simulink model "SOH_second"  (R2025a)
settings: Solver=VariableStepAuto  StartTime=0.0  StopTime=100  RelTol=1e-3
libraries: nesl_utility x7, fl_lib x5, batt_lib x1, spsDiscreteVariableTimeDelayLib x1, BatteryEstimators x1
settings Model: Creator=aassd  LastModifiedBy=aassd

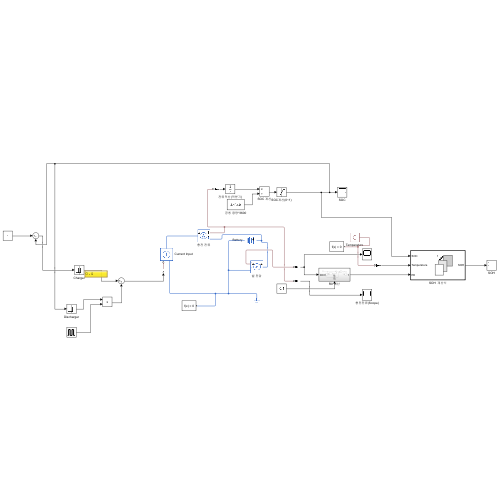
[thumbnail: Simulink's stored preview of the top-level diagram]
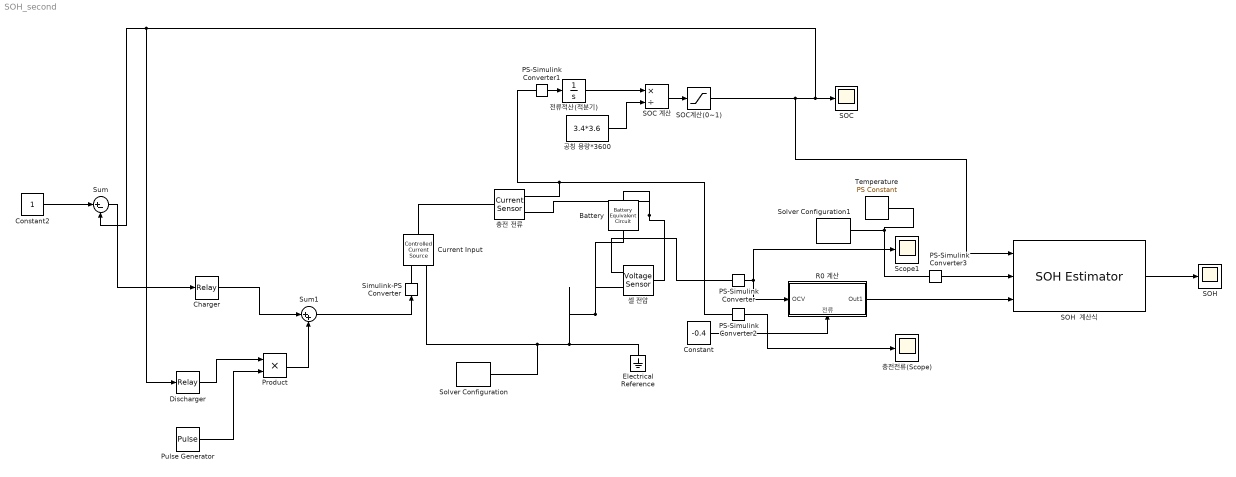
== system SOH_second ==
  Battery : batt_lib/Cells/Battery Equivalent Circuit  BatteryCapacity=3.4 A*hr  ThermalModel=simscape.battery.enum.cells.BatteryThermalModel.ConstantTemperature  ExtrapolationMethod=simscape.enum.extrapolation.linear  SOCBreakpoints=[0, 0.111071, 0.222202, 0.333333, 0.444465, 0.555535, 0.666667, 0.777798, 0.888869]  TemperatureBreakpoints=[273.15, 298.15, 318.15] K  OpenCircuitVoltage=[3.5057, 3.566, 3.6337, 3.7127, 3.9259, 4.0777, 4.1928] V  OpenCircuitVoltageThermal=[4.0405, 4.0578, 4.0648; 3.9374, 3.9475, 3.9556; 3.844, 3.8471, 3.8552; 3.759, 3.7591, 3.7659; 3.671, 3.67, 3.6778; 3.6282, 3.6287, 3.6355; 3.6009, 3.6013, 3.608; 3.5742, 3.5621, 3.5612; 3.4716, 3.3585, 3.3997;] V  VoltageRange=[0, inf] V  HysteresisModel=simscape.battery.enum.cells.HysteresisModel.none  MaximumHysteresisVoltage=[0, 0, 0, 0, 0, 0, 0] V  InstantaneousHysteresisVoltage=[0, 0, 0, 0, 0, 0, 0] V  HysteresisRate=0.1  MaximumHysteresisVoltageThermal=[0, 0, 0; 0, 0, 0; 0, 0, 0; 0, 0, 0; 0, 0, 0; 0, 0, 0; 0, 0, 0] V  InstantaneousHysteresisVoltageThermal=[0, 0, 0; 0, 0, 0; 0, 0, 0; 0, 0, 0; 0, 0, 0; 0, 0, 0; 0, 0, 0] V  HysteresisRateThermal=0.1  ResistanceSOCBreakpoints=[0, 0.111071, 0.222202, 0.333333, 0.444465, 0.555535, 0.666667, 0.777798, 0.888869]  ResistanceTemperatureBreakpoints=[273.15, 298.15, 318.15] K  ResistanceCurrentBreakpoints=[-1, 0, 1] A  CurrentDependence=simscape.battery.enum.cells.CurrentDependence.Disabled  R0=[.0085, .0085, .0087, .0082, .0083, .0085, .0085] Ohm  R0I=[.0117, .0085, .009; .011, .0085, .009; .0114, .0087, .0092; .0107, .0082, .0088; .0107, .0083, .0091; .0113, .0085, .0089; .0116, .0085, .0089] Ohm  R0Thermal=|  R0ThermalI=repmat([.0117, .0085, .009; .011, .0085, .009; .0114, .0087, .0092; .0107, .0082, .0088; .0107, .0083, .0091; .0113, .0085, .0089; .0116, .0085, .0089], 1, 1, 3) Ohm  DischargeR0=[.0085, .0085, .0087, .0082, .0083, .0085, .0085] Ohm  ChargeR0=[.0085, .0085, .0087, .0082, .0083, .0085, .0085] Ohm  ChargeR0Thermal=[.0117, .0085, .009; .011, .0085, .009; .0114, .0087, .0092; .0107, .0082, .0088; .0107, .0083, .0091; .0113, .0085, .0089; .0116, .0085, .0089] Ohm  DischargeR0Thermal=[.0117, .0085, .009; .011, .0085, .009; .0114, .0087, .0092; .0107, .0082, .0088; .0107, .0083, .0091; .0113, .0085, .0089; .0116, .0085, .0089] Ohm  RCPairs=simscape.battery.enum.cells.RCPairs.rc2  R1=[.0029, .0024, .0026, .0016, .0023, .0018, .0017] Ohm  Tau1=[36, 45, 105, 29, 77, 33, 39] s  R2=[.0029, .0024, .0026, .0016, .0023, .0018, .0017] Ohm  Tau2=[36, 45, 105, 29, 77, 33, 39] s  R3=[.0029, .0024, .0026, .0016, .0023, .0018, .0017] Ohm  Tau3=[36, 45, 105, 29, 77, 33, 39] s  R1I=[.0109, .0029, .0013; .0069, .0024, .0012; .0047, .0026, .0013; .0034, .0016, .001; .0033, .0023, .0014; .0033, .0018, .0011; .0028, .0017, .0011] Ohm  Tau1I=[20, 36, 39; 31, 45, 39; 109, 105, 61; 36, 29, 26; 59, 77, 67; 40, 33, 29; 25, 39, 33] s  R2I=[.0109, .0029, .0013; .0069, .0024, .0012; .0047, .0026, .0013; .0034, .0016, .001; .0033, .0023, .0014; .0033, .0018, .0011; .0028, .0017, .0011] Ohm  Tau2I=[20, 36, 39; 31, 45, 39; 109, 105, 61; 36, 29, 26; 59, 77, 67; 40, 33, 29; 25, 39, 33] s  R3I=[.0109, .0029, .0013; .0069, .0024, .0012; .0047, .0026, .0013; .0034, .0016, .001; .0033, .0023, .0014; .0033, .0018, .0011; .0028, .0017, .0011] Ohm  Tau3I=[20, 36, 39; 31, 45, 39; 109, 105, 61; 36, 29, 26; 59, 77, 67; 40, 33, 29; 25, 39, 33] s  DischargeR1=[.0029, .0024, .0026, .0016, .0023, .0018, .0017] Ohm  DischargeTau1=[36, 45, 105, 29, 77, 33, 39] s  ChargeR1=[.0029, .0024, .0026, .0016, .0023, .0018, .0017] Ohm  ChargeTau1=[36, 45, 105, 29, 77, 33, 39] s  DischargeR2=[.0029, .0024, .0026, .0016, .0023, .0018, .0017] Ohm  DischargeTau2=[36, 45, 105, 29, 77, 33, 39] s  ChargeR2=[.0029, .0024, .0026, .0016, .0023, .0018, .0017] Ohm  ChargeTau2=[36, 45, 105, 29, 77, 33, 39] s  DischargeR3=[.0029, .0024, .0026, .0016, .0023, .0018, .0017] Ohm  DischargeTau3=[36, 45, 105, 29, 77, 33, 39] s  ChargeR3=[.0029, .0024, .0026, .0016, .0023, .0018, .0017] Ohm  ChargeTau3=[36, 45, 105, 29, 77, 33, 39] s  R1Thermal=|  Tau1Thermal=|  R2Thermal=|  Tau2Thermal=|  R3Thermal=[0.0001, 0.0001, 0.0001; 0.0001, 0.0001, 0.0001; 0.0001, 0.0001, 0.0001; 0.0001, 0.0001, 0.0001; 0.0001, 0.0001, 0.0001; 0.0001, 0.0001, 0.0001; 0.0001, 0.0001, 0.0001; 0.0001, 0.0001, 0.0001; 0.0001, 0.0001, 0.0001;] Ohm  Tau3Thermal=[0.0001, 0.0001, 0.0001; 0.0001, 0.0001, 0.0001; 0.0001, 0.0001, 0.0001; 0.0001, 0.0001, 0.0001; 0.0001, 0.0001, 0.0001; 0.0001, 0.0001, 0.0001; 0.0001, 0.0001, 0.0001; 0.0001, 0.0001, 0.0001; 0.0001, 0.0001, 0.0001;] s  R1ThermalI=repmat([.0109, .0029, .0013; .0069, .0024, .0012; .0047, .0026, .0013; .0034, .0016, .001; .0033, .0023, .0014; .0033, .0018, .0011; .0028, .0017, .0011], 1, 1, 3) Ohm  Tau1ThermalI=repmat([20, 36, 39; 31, 45, 39; 109, 105, 61; 36, 29, 26; 59, 77, 67; 40, 33, 29; 25, 39, 33], 1, 1, 3) s  R2ThermalI=repmat([.0109, .0029, .0013; .0069, .0024, .0012; .0047, .0026, .0013; .0034, .0016, .001; .0033, .0023, .0014; .0033, .0018, .0011; .0028, .0017, .0011], 1, 1, 3) Ohm  Tau2ThermalI=repmat([20, 36, 39; 31, 45, 39; 109, 105, 61; 36, 29, 26; 59, 77, 67; 40, 33, 29; 25, 39, 33], 1, 1, 3) s  R3ThermalI=repmat([.0109, .0029, .0013; .0069, .0024, .0012; .0047, .0026, .0013; .0034, .0016, .001; .0033, .0023, .0014; .0033, .0018, .0011; .0028, .0017, .0011], 1, 1, 3) Ohm  Tau3ThermalI=repmat([20, 36, 39; 31, 45, 39; 109, 105, 61; 36, 29, 26; 59, 77, 67; 40, 33, 29; 25, 39, 33], 1, 1, 3) s  DischargeR1Thermal=[.0109, .0029, .0013; .0069, .0024, .0012; .0047, .0026, .0013; .0034, .0016, .001; .0033, .0023, .0014; .0033, .0018, .0011; .0028, .0017, .0011] Ohm  DischargeTau1Thermal=[20, 36, 39; 31, 45, 39; 109, 105, 61; 36, 29, 26; 59, 77, 67; 40, 33, 29; 25, 39, 33] s  ChargeR1Thermal=[.0109, .0029, .0013; .0069, .0024, .0012; .0047, .0026, .0013; .0034, .0016, .001; .0033, .0023, .0014; .0033, .0018, .0011; .0028, .0017, .0011] Ohm  ChargeTau1Thermal=[20, 36, 39; 31, 45, 39; 109, 105, 61; 36, 29, 26; 59, 77, 67; 40, 33, 29; 25, 39, 33] s  DischargeR2Thermal=[.0109, .0029, .0013; .0069, .0024, .0012; .0047, .0026, .0013; .0034, .0016, .001; .0033, .0023, .0014; .0033, .0018, .0011; .0028, .0017, .0011] Ohm  DischargeTau2Thermal=[20, 36, 39; 31, 45, 39; 109, 105, 61; 36, 29, 26; 59, 77, 67; 40, 33, 29; 25, 39, 33] s  ChargeR2Thermal=[.0109, .0029, .0013; .0069, .0024, .0012; .0047, .0026, .0013; .0034, .0016, .001; .0033, .0023, .0014; .0033, .0018, .0011; .0028, .0017, .0011] Ohm  ChargeTau2Thermal=[20, 36, 39; 31, 45, 39; 109, 105, 61; 36, 29, 26; 59, 77, 67; 40, 33, 29; 25, 39, 33] s  DischargeR3Thermal=[.0109, .0029, .0013; .0069, .0024, .0012; .0047, .0026, .0013; .0034, .0016, .001; .0033, .0023, .0014; .0033, .0018, .0011; .0028, .0017, .0011] Ohm  DischargeTau3Thermal=[20, 36, 39; 31, 45, 39; 109, 105, 61; 36, 29, 26; 59, 77, 67; 40, 33, 29; 25, 39, 33] s  ChargeR3Thermal=[.0109, .0029, .0013; .0069, .0024, .0012; .0047, .0026, .0013; .0034, .0016, .001; .0033, .0023, .0014; .0033, .0018, .0011; .0028, .0017, .0011] Ohm  ChargeTau3Thermal=[20, 36, 39; 31, 45, 39; 109, 105, 61; 36, 29, 26; 59, 77, 67; 40, 33, 29; 25, 39, 33] s  SelfDischargeResistor=simscape.battery.enum.cells.BatteryEnable.Disabled  SelfDischargeR=7e3 Ohm  SelfDischargeRThermal=[8000, 7000, 6000] Ohm  CyclingAgingMethod=simscape.battery.enum.cells.CyclingAgingMethod.disabled  CycleCalculationMethod=simscape.battery.enum.cells.CycleCalculationMethod.EquivalentCycles  NumDisCycles=100  OCVChange=0  R0Change=0  CapacityChange=0  SelfDischargeRChange=0  R1Change=0  R2Change=0  R3Change=0  NumDisCyclesBreakpoints=[1, 100, 200, 300, 400]  AgingTemperatureBreakpoints=[273.15, 298.15, 318.15] K  AgingCurrentBreakpoints=[-.1, -.5, -5] A  OCVChangeVec=[0, 0, 0, 0]  OCVChangeThermal=[0, 0; 0, 0; 0, 0; 0, 0]  R0ChangeVec=[0, 0, 0, 0]  R0ChangeThermal=[0.175588, 0.109515, 0.101823; 0.184275, 0.109516, 0.106861; 0.193050, 0.114730, 0.111949; 0.201825, 0.119945, 0.117038; 0.210600, 0.125160, 0.122126]  R0ChangeThermalI=repmat(0, 4, 3, 3)  R0CyclingChangeInitialTarget=[0.17558774966346, 0.104352149971663, 0.101822886, 0.1, 0.1]  CapacityChangeVec=[0, 0, 0, 0]  CapacityChangeThermal=[3.3026, 3.30259, 3.30258; 3.0002, 3.00019, 2.97540; 2.9354, 2.93539, 2.87640; 2.8382, 2.83819, 2.72790; 2.7734, 2.77339, 2.62890]  CapacityChangeThermalI=repmat(0, 4, 3, 3)  CapacityCyclingChangeInitialTarget=[3.3026, 3.30259, 3.30258 ,0.1, 0.1]  SelfDischargeRChangeVec=[0, 0, 0, 0]  SelfDischargeRChangeThermal=[0, 0; 0, 0; 0, 0; 0, 0]  SelfDischargeRChangeThermalI=repmat(0, 4, 2, 3)  SelfDischargeRCyclingChangeInitialTarget=0  R1ChangeVec=[0, 0, 0, 0]  R1ChangeThermal=[0.0749,0.0309,0.0236;0.0786,0.0324,0.0248;0.0823,0.0340,0.0260;0.0860,0.0355,0.0272;0.0898,0.0371,0.0283]  R1ChangeThermalI=repmat(0, 4, 3, 3)  R1CyclingChangeInitialTarget=[0.0749, 0.0309, 0.0236, 0.1, 0.1]  R2ChangeVec=[0, 0, 0, 0]  R2ChangeThermal=[0.2210,0.2050,0.5240;0.2319,0.2151,0.5497;0.2429,0.2252,0.5758;0.2540,0.2355,0.6020;0.2650,0.2547,0.6282]  R2ChangeThermalI=repmat(0, 4, 3, 3)  R2CyclingChangeInitialTarget=[0.2210, 0.2050, 0.5240, 0.1, 0.1]  R3ChangeVec=[0, 0, 0, 0]  R3ChangeThermal=[0, 0, 0; 0, 0, 0; 0, 0, 0; 0, 0, 0; 0, 0, 0]  R3ChangeThermalI=repmat(0, 4, 2, 3)  R3CyclingChangeInitialTarget=[0, 0, 0, 0, 0]  CalendarAgeResistance=simscape.battery.enum.cells.BatteryEnable.Disabled  CalendarAgeCapacity=simscape.battery.enum.cells.BatteryEnable.Disabled  CalendarAgingMethod=simscape.battery.enum.cells.CalendarAgingMethod.equation  StorageVariable=simscape.battery.enum.cells.StorageVariable.OCV  OCVDuringStorage=0.9  SOCDuringStorage=0.6  StorageTimeIntervals=[0] d  StorageTemperatures=[273] K  ResistanceScalingOCV=2.2134e6  ResistanceScalingOCVOffset=1.632e6  ResistanceExponentialIncrease=0.515833569 V  ResistanceTimeExponent=0.75  ResistanceAgeTemperatureBreakpoints=[273.15, 298.15, 323.15] K  ResistanceAgeTimeBreakpoints=[0, 90, 180, 270] d  PercentResistanceChange=[0, 0, 0]  ResistanceTimeBreakpoints=100 d  PercentResistanceChangeThermal=[0, 0, 0; 0, 0, 0; 0, 0, 0; 0, 0, 0]  CapacityScalingOCV=1.5097e07  CapacityScalingOCVOffset=8.3625e06  CapacityExponentialIncrease=0.6011 V  CapacityTimeExponent=0.75  CapacityAgeTemperatureBreakpoints=[273.15, 298.15, 323.15] K  CapacityAgeTimeBreakpoints=[0, 90, 180, 270] d  PercentCapacityChange=[0, 0, 0]  CapacityTimeBreakpoints=100 d  PercentCapacityChangeThermal=[0, 0, 0; 0, 0, 0; 0, 0, 0; 0, 0, 0]  SimulationTemperature=298.15 K  BatteryThermalMass=100 J/K  NumThermalModels=6  ThermalConductivityZ=18 W/(K*m)  CrossSectionalAreaXY=3.5e-4 m^2  Height=0.07 m  ReversibleHeatModel=simscape.battery.enum.cells.ReversibleHeatModel.Disabled  EntropicCoefficient=[0, 0, 0, 0, 0, 0, 0] mV/K  CurrentDirectionality=simscape.battery.enum.cells.BatteryEnable.Disabled  stateOfCharge_specify=on  stateOfCharge_priority=High  stateOfCharge=0  stateOfCharge_nominal_specify=off  stateOfCharge_nominal_value=1  stateOfCharge_nominal_unit=1  batteryVoltage_specify=on  batteryVoltage_priority=None  batteryVoltage=3.4 V  batteryVoltage_nominal_specify=on  batteryVoltage_nominal_value=3.7  batteryVoltage_nominal_unit=V  batteryCurrent_specify=off  batteryCurrent_priority=None  batteryCurrent=0 A  batteryCurrent_nominal_specify=off  batteryCurrent_nominal_value=1  batteryCurrent_nominal_unit=A  numCycles_specify=off  numCycles_priority=High  numCycles=0  numCycles_nominal_specify=off  numCycles_nominal_value=1  numCycles_nominal_unit=1  batteryTemperature_specify=off  batteryTemperature_priority=High  batteryTemperature=298.15 K  batteryTemperature_nominal_specify=off  batteryTemperature_nominal_value=1  batteryTemperature_nominal_unit=K  hysteresisState_specify=off  hysteresisState_priority=High  hysteresisState=0  hysteresisState_nominal_specify=off  hysteresisState_nominal_value=1  hysteresisState_nominal_unit=1  isExothermFaulted_specify=off  isExothermFaulted_priority=None  isExothermFaulted=0  isExothermFaulted_nominal_specify=off  isExothermFaulted_nominal_value=1  isExothermFaulted_nominal_unit=1  reactionHeatRate_specify=off  reactionHeatRate_priority=None  reactionHeatRate=0 W  reactionHeatRate_nominal_specify=off  reactionHeatRate_nominal_value=1  reactionHeatRate_nominal_unit=W  reactionExtent_specify=off  reactionExtent_priority=None  reactionExtent=0  reactionExtent_nominal_specify=off  reactionExtent_nominal_value=1  reactionExtent_nominal_unit=1
      R0Thermal=|
      | [0.1321, 0.1056, 0.0769; 0.1227, 0.1035, 0.0765;
      | 0.1069, 0.1032, 0.0763;
      | 0.1087, 0.1033, 0.0776;
      | 0.1154, 0.1041, 0.0771;
      | 0.1170, 0.1043, 0.0771;
      | 0.1155, 0.1043, 0.0771;
      | 0.1040, 0.1043, 0.0771;
      | 0.1089, 0.1046, 0.0755] Ohm
      R1Thermal=|
      | [0.0268, 0.0173, 0.0106; 0.0368, 0.0209, 0.0154; 0.0288, 0.0172, 0.0126;
      | 0.0309, 0.0160, 0.0118;
      | 0.0490, 0.0354, 0.0265;
      | 0.0499, 0.0205, 0.0265;
      | 0.0456, 0.0309, 0.0179; 0.0279, 0.0234, 0.0090;
      | 0.0346, 0.0177, 0.0099] Ohm
      Tau1Thermal=|
      | [11.1032, 29.4916, 13.0203;
      | 41.6392, 50.3057, 44.4809;
      | 31.8702, 36.7367, 31.2302;
      | 30.5023, 20.2959, 22.4176;
      | 28.8031, 36.3713, 48.2173;
      | 31.3147, 35.1393, 25.4136;
      | 34.2325, 27.2197, 19.334;
      | 33.7415, 24.6218, 17.5816;
      | 35.7035, 22.7467, 18.3252
      | ] s
      R2Thermal=|
      | [4.3413, 0.7404, 1.1858;
      | 4.3413, 0.7404, 1.1858;
      | 0.2169, 0.1906, 0.2428;
      | 0.1282, 0.0892, 0.2428;
      | 0.0760, 0.0768, 0.0850;
      | 0.1070, 0.1151, 0.1204;
      | 0.1473, 0.2049, 0.3968;
      | 0.2062, 0.4119, 0.4750;
      | 0.2785, 0.4363, 0.5223
      | ] Ohm
      Tau2Thermal=|
      | [1223.8, 4578.136, 9123.614;
      | 1294.722, 2067.605, 3124.982;
      | 808.9907, 1093.649, 1297.938;
      | 485.3542, 659.0507, 916.6587;
      | 547.9316, 651.394, 713.2342;
      | 639.6711, 1000.979, 2358.11;
      | 897.0311, 2167.331, 2765.437;
      | 1055.746, 2224.096, 2581.318;
      | 1893.941, 2140.673, 2547.088
      | ] s
      settings: InternalSimscapePortConfiguration="{\"Bottom\":[{\"id\":\"n\",\"label\":\"-\",\"type\":\"foundation.electrical.electrical\"}],\"Left\":[],\"Right\":[],\"Top\":[{\"id\":\"p\",\"label\":\"+\",\"type\":\"foundation.electrical.electrical\"}]}"
  Charger : Relay  OnSwitchValue=0.9  OffSwitchValue=0  OnOutputValue=0.4
  Constant : Constant  Value=-0.4
  Constant2 : Constant
  Current Input : fl_lib/Electrical/Electrical Sources/Controlled Current Source
  Discharger : Relay  OnSwitchValue=1  OffSwitchValue=0.1  OnOutputValue=-0.4
  Electrical Reference : fl_lib/Electrical/Electrical Elements/Electrical Reference
  PS-Simulink Converter{,1..3} (4 alike) : nesl_utility/PS-Simulink Converter  PhysicalDomain=network_engine_domain  SubClassName=ps_output  LeftPortType=input  RightPortType=output  PseudoPeriodic=off  Frequencies=[]  VectorFormat=inherit  Unit=inherit  AffineConversion=off
  Product : Product
  Pulse Generator : DiscretePulseGenerator  PulseType=Time based  PulseWidth=50
  R0 계산 : Subsystem
      settings: PortSchema="{\"entries\":[{\"content\":{\"sides\":[{\"content\":{\"connectorIds\":[\"In1\"]},\"type\":\"ConnectorPlacement.EquallySpacedRectSide\",\"uuid\":\"284c04bd-4081-43f1-9d69-2474095be116\"},{\"content\":{\"connectorIds\":[\"Out1\"],\"side\":\"RIGHT\"},\"type\":\"ConnectorPlacement.EquallySpacedRectSide\",\"uuid\":\"f0711672-b87d-4fdd-b10d-18b7afa3813d\"},{\"content\":{\"side\":\"TOP\"},\"type\":\"ConnectorPlacement.EquallySpacedRectSide\",\"uuid\":\"94732b66-d90d-4c43-963d-8f72a09e0221\"},{\"content\":{\"connectorIds\":[\"In2\"],\"side\":\"BOTTOM\"},\"type\":\"ConnectorPlacement.EquallySpacedRectSide\",\"uuid\":\"99cfaf90-d72b-4a53-a397-ebd1f88ec8e8\"}]},\"type\":\"ConnectorPlacement.EquallySpacedConnector\",\"uuid\":\"2fcb15ae-0bbd-4ef2-904b-0d1e2d5bb78c\"}],\"packageUris\":[\"http://schema.mathworks.com/mf0/Connector/R2020b\"],\"version\":\"1.0\"}"
  SOC : Scope
      settings: ActiveDisplayYMinimum=-1.9003374212908724  ActiveDisplayYMaximum=0.6794811319877232
  SOC 계산 : Product  Inputs=*/
  SOC계산(0~1) : Saturate  UpperLimit=1  LowerLimit=0
  SOH : Scope
      settings: ActiveDisplayYMinimum=-0.8984015366778646  ActiveDisplayYMaximum=1.7206339658692529  DataLoggingVariableName=ScopeData3
  SOH  계산식 : BatteryEstimators/SOH Estimator  SOC_vec=[0, 0.111071, 0.222202, 0.333333, 0.444465, 0.555535, 0.666667, 0.777798, 0.888869]  T_vec=[273, 298, 318]  R0_new_mat=|  R0_EOL_mat=|  DataType=Inherit: auto
      R0_new_mat=|
      | [0.1321, 0.1056, 0.0769; 0.1227, 0.1035, 0.0765;
      | 0.1069, 0.1032, 0.0763;
      | 0.1087, 0.1033, 0.0776;
      | 0.1154, 0.1041, 0.0771;
      | 0.1170, 0.1043, 0.0771;
      | 0.1155, 0.1043, 0.0771;
      | 0.1040, 0.1043, 0.0771;
      | 0.1089, 0.1046, 0.0755]
      R0_EOL_mat=|
      | [0.251689, 0.146491, 0.150106;
      |  0.242368, 0.141066, 0.144547;
      | 0.233048, 0.135641, 0.138988;
      | 0.223727, 0.130216, 0.133429;
      |  0.214406, 0.12479,  0.12787;
      | 0.214397, 0.124786, 0.127865;
      | 0.223718, 0.130211, 0.133424;
      | 0.233039, 0.135636, 0.138983;
      | 0.24236, 0.141061, 0.144542]
      settings: LibrarySourceBlock=batt_sl_lib/Estimators/SOH Estimator
  Scope1 : Scope
      settings: ActiveDisplayYMinimum=3.9522947930051937  ActiveDisplayYMaximum=4.2293088325990871
  Simulink-PS Converter : nesl_utility/Simulink-PS Converter  PhysicalDomain=network_engine_domain  SubClassName=ps_input  LeftPortType=input  RightPortType=output  PseudoPeriodic=off  Frequencies=[]  NoiseDistribution=none  NoiseParameters=[]  Unit=1  AffineConversion=off  FilteringAndDerivatives=provide  SimscapeFilterOrder=1  InputFilterTimeConstant=0.001  UdotUserProvided=0
  Solver Configuration : nesl_utility/Solver Configuration  PhysicalDomain=network_engine_domain  SubClassName=solver  LeftPortType=input  RightPortType=generic  Tones=[]  Harmonics=[]  SimulateNoise=off  Profile=off  UseLocalSampling=off  EnableSwitchedLinearOptims=on  FrequencyDomain=off  UseCCode=off  RelTol=0.001  AbsTol=0.001  MinStep=1e-09  ToWorkspace=off  RevertToSquareIcSolve=off  NumHomotopyIterations=100  PhasorMode=off  PhasorModeNumHarmonics=1  ConsistencySolver=NEWTON_XTOL_AFTER_FTOL  IndexReductionMethod=DerivativeReplacement  DoDC=off  ResidualTolerance=1e-09  ConsistencyTolSource=GLOBAL  ConsistencyAbsTol=0.001  ConsistencyRelTol=0.001  ConsistencyTolFactor=0.001  UseLocalSolver=off  LocalSolverChoice=NE_BACKWARD_EULER_ADVANCER  ResolveIndetEquations=on  FunctionEvalNumThread=1  LocalSolverSampleTime=0.001  DoFixedCost=off  MaxNonlinIter=3  MaxModeIter=2  ComputeImpulses=off  ImpulseIterations=2  LinearAlgebra=auto  LinearAlgebraNumThread=0  EquationFormulation=NE_TIME_EF  DelaysMemoryBudget=1024  AutomaticFiltering=on  FilteringTimeConstant=0.001  PartitionStorageMethod=AS_NEEDED  PartitionMemoryBudget=1024  PartitionMethod=ROBUST  MultibodyUseLocalSolver=off  MultibodyLocalSolverChoice=ODE1  MultibodyLocalSolverSampleTime=0.001
  Solver Configuration1 : nesl_utility/Solver Configuration  PhysicalDomain=network_engine_domain  SubClassName=solver  LeftPortType=input  RightPortType=generic  Tones=[]  Harmonics=[]  SimulateNoise=off  Profile=off  UseLocalSampling=off  EnableSwitchedLinearOptims=on  FrequencyDomain=off  UseCCode=off  RelTol=0.001  AbsTol=0.001  MinStep=1e-09  ToWorkspace=off  RevertToSquareIcSolve=off  NumHomotopyIterations=100  PhasorMode=off  PhasorModeNumHarmonics=1  ConsistencySolver=NEWTON_XTOL_AFTER_FTOL  IndexReductionMethod=DerivativeReplacement  DoDC=off  ResidualTolerance=1e-09  ConsistencyTolSource=GLOBAL  ConsistencyAbsTol=0.001  ConsistencyRelTol=0.001  ConsistencyTolFactor=0.001  UseLocalSolver=off  LocalSolverChoice=NE_BACKWARD_EULER_ADVANCER  ResolveIndetEquations=on  FunctionEvalNumThread=1  LocalSolverSampleTime=0.001  DoFixedCost=off  MaxNonlinIter=3  MaxModeIter=2  ComputeImpulses=off  ImpulseIterations=2  LinearAlgebra=auto  LinearAlgebraNumThread=0  EquationFormulation=NE_TIME_EF  DelaysMemoryBudget=1024  AutomaticFiltering=on  FilteringTimeConstant=0.001  PartitionStorageMethod=AS_NEEDED  PartitionMemoryBudget=1024  PartitionMethod=ROBUST  MultibodyUseLocalSolver=off  MultibodyLocalSolverChoice=ODE1  MultibodyLocalSolverSampleTime=0.001
  Sum : Sum  Inputs=|+-
  Sum1 : Sum  Inputs=|++
  Temperature : fl_lib/Physical Signals/Sources/PS Constant  constant=273.15 K
  공칭 용량*3600 : Constant  Value=3.4*3.6
  셀 전압 : fl_lib/Electrical/Electrical Sensors/Voltage Sensor
  전류적산(적분기) : Integrator  InitialCondition=0.34*3.6
  충전 전류 : fl_lib/Electrical/Electrical Sensors/Current Sensor
  충전전류(Scope) : Scope
      settings: ActiveDisplayYMinimum=-1  ActiveDisplayYMaximum=1  DataLoggingVariableName=ScopeData2
  wires:
  SOC 계산/1 -> SOC계산(0~1)/1
  공칭 용량*3600/1 -> SOC 계산/2
  PS-Simulink Converter1/1 -> 전류적산(적분기)/1
  PS-Simulink Converter/1 -> R0 계산/1(OCV), Scope1/1
  PS-Simulink Converter2/1 -> 충전전류(Scope)/1
  SOH  계산식/1 -> SOH/1
  전류적산(적분기)/1 -> SOC 계산/1
  Constant2/1 -> Sum/1
  Sum/1 -> Charger/1
  SOC계산(0~1)/1 -> SOH  계산식/1, Sum/2, Discharger/1, SOC/1
  R0 계산/1(Out1) -> SOH  계산식/3
  PS-Simulink Converter3/1 -> SOH  계산식/2
  Charger/1 -> Sum1/1
  Pulse Generator/1 -> Product/2
  Discharger/1 -> Product/1
  Product/1 -> Sum1/2
  Sum1/1 -> Simulink-PS Converter/1
  Constant/1 -> R0 계산/2(전류)
  connections:
  충전 전류/LConn1 -- Current Input/LConn1
  Battery/RConn1 -- Solver Configuration/RConn1 -- Current Input/RConn2 -- Electrical Reference/LConn1 -- 셀 전압/RConn2
  셀 전압/RConn1 -- PS-Simulink Converter/LConn1
  Temperature/RConn1 -- Solver Configuration1/RConn1 -- PS-Simulink Converter3/LConn1
  Simulink-PS Converter/RConn1 -- Current Input/RConn1
  충전 전류/RConn2 -- 셀 전압/LConn1 -- Battery/LConn1
  충전 전류/RConn1 -- PS-Simulink Converter1/LConn1 -- PS-Simulink Converter2/LConn1

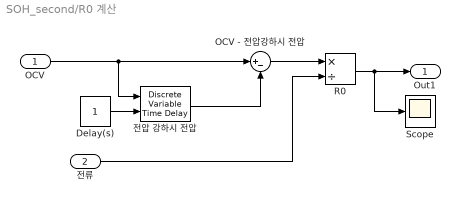
== system SOH_second/R0 계산 ==
  OCV : Inport
  전류 : Inport  Port=2
  Delay(s) : Constant
  OCV - 전압강하시 전압 : Sum  Inputs=|+-
  R0 : Product  Inputs=*/
  Scope : Scope
      settings: ActiveDisplayYMinimum=-0.31375855792624469  ActiveDisplayYMaximum=0.52517111589319021  DataLoggingVariableName=ScopeData4
  전압 강하시 전압 : spsDiscreteVariableTimeDelayLib/Discrete Variable Time Delay  MaxDelay=1  InitialValue=0  Ts=50e-6  DFT=on
      settings: LibrarySourceBlock=|
      | sps_lib/Control/Discrete Variable
      | Time Delay
  Out1 : Outport
  wires:
  OCV/1 -> 전압 강하시 전압/1, OCV - 전압강하시 전압/1
  전류/1 -> R0/2
  OCV - 전압강하시 전압/1 -> R0/1
  R0/1 -> Scope/1, Out1/1
  Delay(s)/1 -> 전압 강하시 전압/2
  전압 강하시 전압/1 -> OCV - 전압강하시 전압/2
